simulink model "Task4"  (R2021a)
settings: Solver=FixedStepDiscrete  StartTime=0.0  StopTime=10.0  RelTol=1e-3  EnableMultiTasking=on
settings Model: Creator=Alaa  LastModifiedBy=Alaa
settings DataIOCC: ReturnWorkspaceOutputs=off
settings OptimizationCC: DefaultParameterBehavior=Inlined  InlineInvariantSignals=on  EnableMemcpy=off  LifeSpan=1  EfficientTunableParamExpr=on
settings DebuggingCC: UnderspecifiedInitializationDetection=Classic  MergeDetectMultiDrivingBlocksExec=none  SFMachineParentedDataDiag=warning  ArithmeticOperatorsInVariantConditions=warning
settings ModelReferenceCC: PropagateSignalLabelsOutOfModel=off
settings SFSimCC: MATLABDynamicMemAlloc=off  CustomCodeUndefinedFunction=UseInterfaceOnly
settings RTWCC: SystemTargetFile=ert.tlc  GenCodeOnly=on  TemplateMakefile=ert_default_tmf  GenerateReport=on  IncludeHyperlinkInReport=on  LaunchReport=on  GenerateTraceInfo=on  GenerateTraceReport=on  GenerateTraceReportSl=on  GenerateTraceReportSf=on  GenerateTraceReportEml=on
settings CodeAppCC: ForceParamTrailComments=on  IgnoreCustomStorageClasses=off  OperatorAnnotations=on  SimulinkDataObjDesc=on  SFDataObjDesc=on  MATLABFcnDesc=on  InsertBlockDesc=on  StateflowObjectComments=on  MATLABSourceComments=on
settings ERTTargetCC: MultiwordLength=2048  GenerateSampleERTMain=on  InlinedParameterPlacement=NonHierarchical  ERTCustomFileTemplate=example_file_process.tlc

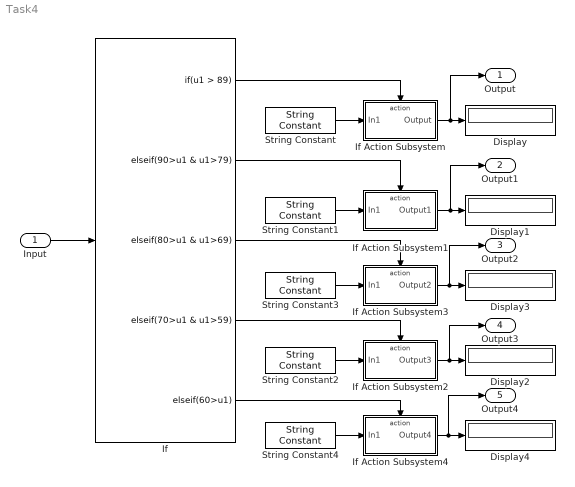
== system Task4 ==
  Input : Inport
  Display{,1..4} (5 alike) : Display
  If : If  IfExpression=u1 > 89  ElseIfExpressions=90>u1 & u1>79, 80>u1 & u1>69, 70>u1 & u1>59, 60>u1  ShowElse=off
  If Action Subsystem : Subsystem  TreatAsAtomicUnit=on
  If Action Subsystem1 : Subsystem  TreatAsAtomicUnit=on
  If Action Subsystem2 : Subsystem  TreatAsAtomicUnit=on
  If Action Subsystem3 : Subsystem  TreatAsAtomicUnit=on
  If Action Subsystem4 : Subsystem  TreatAsAtomicUnit=on
  String Constant : StringConstant  String="\"Excellent\""
  String Constant1 : StringConstant  String="\"Very good\""
  String Constant2 : StringConstant  String="\"Passable\""
  String Constant3 : StringConstant  String="\"Good\""
  String Constant4 : StringConstant  String="\"Failure\""
  Output : Outport  OutDataTypeStr=string
  Output1 : Outport  Port=2  OutDataTypeStr=string
  Output2 : Outport  Port=3  OutDataTypeStr=string
  Output3 : Outport  Port=4  OutDataTypeStr=string
  Output4 : Outport  Port=5  OutDataTypeStr=string
  wires:
  String Constant/1 -> If Action Subsystem/1(In1)
  If/1 -> If Action Subsystem/Action
  If Action Subsystem/1(Output) -> Output/1, Display/1
  If Action Subsystem1/1(Output1) -> Output1/1, Display1/1
  String Constant1/1 -> If Action Subsystem1/1(In1)
  If Action Subsystem2/1(Output3) -> Output3/1, Display2/1
  String Constant2/1 -> If Action Subsystem2/1(In1)
  If Action Subsystem3/1(Output2) -> Output2/1, Display3/1
  String Constant3/1 -> If Action Subsystem3/1(In1)
  If Action Subsystem4/1(Output4) -> Output4/1, Display4/1
  String Constant4/1 -> If Action Subsystem4/1(In1)
  If/2 -> If Action Subsystem1/Action
  If/3 -> If Action Subsystem3/Action
  If/4 -> If Action Subsystem2/Action
  If/5 -> If Action Subsystem4/Action
  Input/1 -> If/1

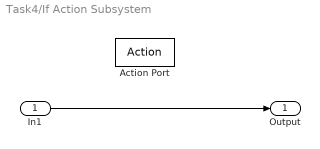
== system Task4/If Action Subsystem ==
  In1 : Inport
  Action Port : ActionPort  ActionPortLabel=if(u1 > 89)
  Output : Outport
  wires:
  In1/1 -> Output/1

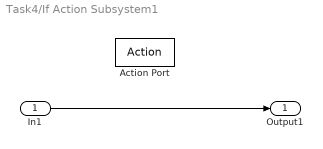
== system Task4/If Action Subsystem1 ==
  In1 : Inport
  Action Port : ActionPort  ActionPortLabel=elseif(90>u1 & u1>79)
  Output1 : Outport
  wires:
  In1/1 -> Output1/1

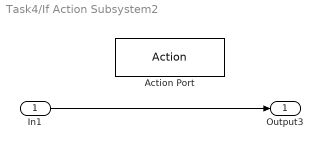
== system Task4/If Action Subsystem2 ==
  In1 : Inport
  Action Port : ActionPort  ActionPortLabel=elseif( 70>u1 & u1>59)
  Output3 : Outport
  wires:
  In1/1 -> Output3/1

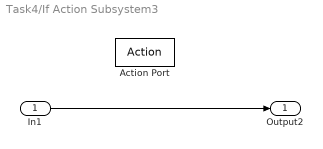
== system Task4/If Action Subsystem3 ==
  In1 : Inport
  Action Port : ActionPort  ActionPortLabel=elseif( 80>u1 & u1>69)
  Output2 : Outport
  wires:
  In1/1 -> Output2/1

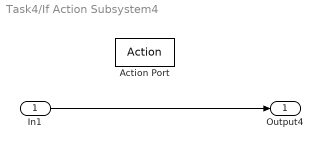
== system Task4/If Action Subsystem4 ==
  In1 : Inport
  Action Port : ActionPort  ActionPortLabel=elseif( 60>u1)
  Output4 : Outport
  wires:
  In1/1 -> Output4/1
